simulink model "lecture8_simpleex"  (Simulink 7.1)
settings: Solver=FixedStepDiscrete  StartTime=0.0  StopTime=Inf  RelTol=1e-3
settings Model: Creator=pit  LastModifiedBy=pit

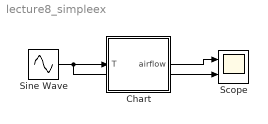
== system lecture8_simpleex ==
  Chart : Stateflow chart
  Scope : Scope  NumInputPorts=2
      settings: TimeRange=300  YMin=0~-5  YMax=1~5
  Sine Wave : Sin  Amplitude=25  Frequency=0.1  SampleTime=0
  wires:
  Chart/1(airflow) -> Scope/1
  Sine Wave/1 -> Chart/1(T), Scope/2

== stateflow chart Chart ==
  state Off
    entry: airflow=0
  state On
    entry: airflow=1
  (default) -> Off
  Off -> On : [T>20]
  On -> Off : [T<10]
  data: airflow output double; T input double
